simulink model "Example9and10"  (R2023b)
settings: Solver=VariableStepAuto  StartTime=0.0  StopTime=15.0  RelTol=1e-3
settings Model: Creator=ray  LastModifiedBy=ray

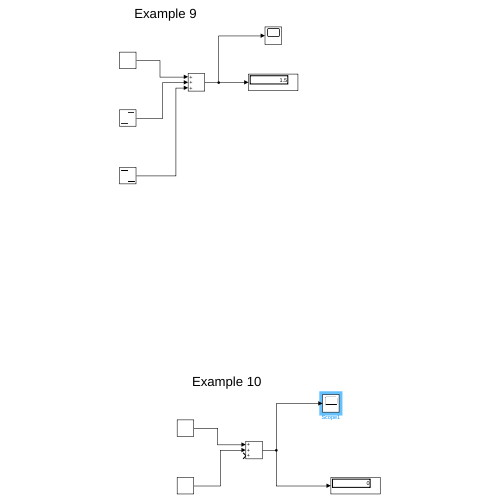
[thumbnail: Simulink's stored preview of the top-level diagram]
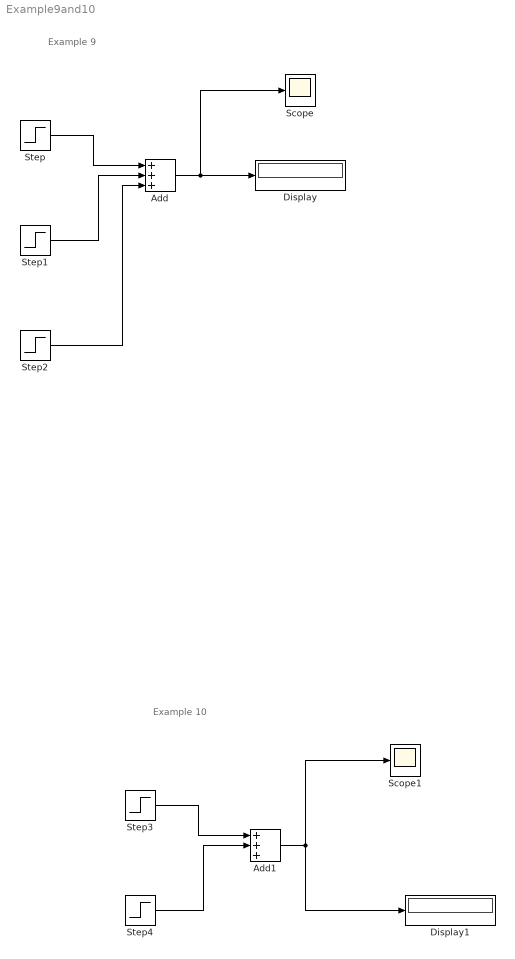
== system Example9and10 ==
  note: Example 9
  note: Example 10
  Add : Sum  Inputs=+++
  Add1 : Sum  Inputs=+++
  Display : Display
  Display1 : Display
  Scope : Scope
  Scope1 : Scope
  Step : Step  Time=5  SampleTime=0
  Step1 : Step  Time=10  SampleTime=0
  Step2 : Step  Time=2  After=-0.5  SampleTime=0
  Step3 : Step  Time=5  SampleTime=0
  Step4 : Step  Time=10  After=-1  SampleTime=0
  wires:
  Step/1 -> Add/1
  Step1/1 -> Add/2
  Add/1 -> Scope/1, Display/1
  Step2/1 -> Add/3
  Step4/1 -> Add1/2
  Add1/1 -> Scope1/1, Display1/1
  Step3/1 -> Add1/1
